simulink model "window_counter_prove"  (R2014b)
settings: Solver=FixedStepDiscrete  StartTime=0.0  StopTime=10.0  FixedStep=0.01  RelTol=1e-3
undefined symbols (not defined in the file): sldvsubsys
libraries: simulink x6, sldvlib x4
settings Model: ModifiedByFormat=Natasha  Creator=Natasha  LastModifiedBy=Natasha
settings DebuggingCC: UnderspecifiedInitializationDetection=Classic  MergeDetectMultiDrivingBlocksExec=none

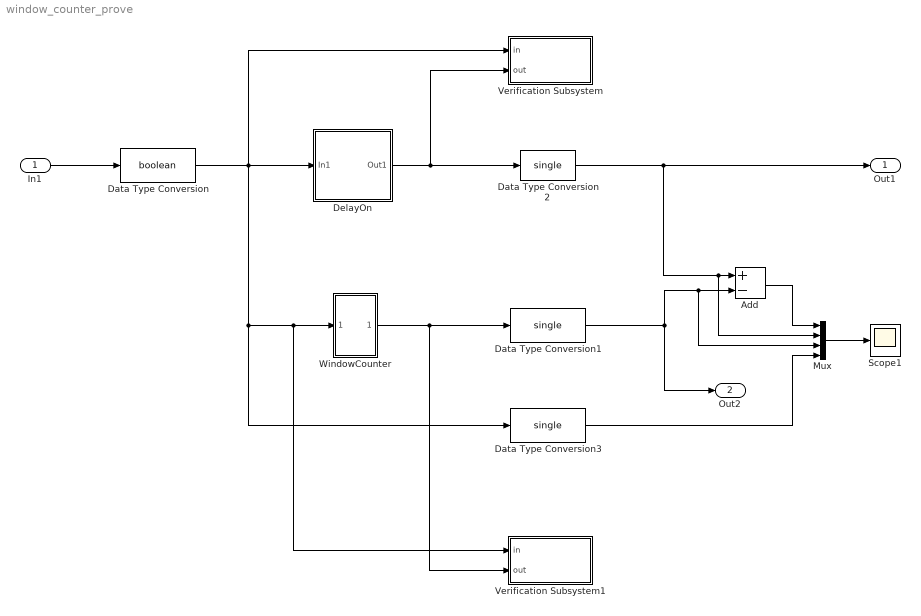
== system window_counter_prove ==
  In1 : Inport
  Add : Sum  Inputs=+-
  Data Type Conversion : DataTypeConversion  OutDataTypeStr=boolean
  Data Type Conversion1 : DataTypeConversion  OutDataTypeStr=single
  Data Type Conversion2 : DataTypeConversion  OutDataTypeStr=single
  Data Type Conversion3 : DataTypeConversion  OutDataTypeStr=single
  DelayOn : Subsystem
  Mux : Mux
  Scope1 : Scope
  Verification Subsystem : Subsystem  Tag=VerificationSubsystem  DisableCoverage=on  LoadFcn=sldvsubsys('check')  TreatAsAtomicUnit=on  SimViewingDevice=on  mask(VerificationSubsystem){}
      mask init:
      | sldvsubsys('maskInit');
      settings: CopyFcn=sldvsubsys('copy');  OpenFcn=open_system(gcb,'force');
      settings: PreSaveFcn=|
      | set_param(gcb,'SimViewingDevice','on');
      | sldvsubsys('check');
      mask Help: helpview(fullfile(docroot,'toolbox','sldv','sldv.map'),'verificationsubsystem')
      mask Display: image(imread('sldvicon_versubsys.png','BackGroundColor',[1 1 1]),'center');
  Verification Subsystem1 : Subsystem  Tag=VerificationSubsystem  DisableCoverage=on  LoadFcn=sldvsubsys('check')  TreatAsAtomicUnit=on  SimViewingDevice=on  mask(VerificationSubsystem){}
      mask init:
      | sldvsubsys('maskInit');
      settings: CopyFcn=sldvsubsys('copy');  OpenFcn=open_system(gcb,'force');
      settings: PreSaveFcn=|
      | set_param(gcb,'SimViewingDevice','on');
      | sldvsubsys('check');
      mask Help: helpview(fullfile(docroot,'toolbox','sldv','sldv.map'),'verificationsubsystem')
      mask Display: image(imread('sldvicon_versubsys.png','BackGroundColor',[1 1 1]),'center');
  WindowCounter : Subsystem
  Out1 : Outport
  Out2 : Outport  Port=2
  wires:
  DelayOn/1(Out1) -> Data Type Conversion2/1, Verification Subsystem/2(out)
  Add/1 -> Mux/1
  Data Type Conversion1/1 -> Out2/1, Mux/3, Add/2
  Data Type Conversion2/1 -> Mux/2, Add/1, Out1/1
  Mux/1 -> Scope1/1
  In1/1 -> Data Type Conversion/1
  WindowCounter/1(Out1) -> Verification Subsystem1/2(out), Data Type Conversion1/1
  Data Type Conversion3/1 -> Mux/4
  Data Type Conversion/1 -> Data Type Conversion3/1, Verification Subsystem1/1(in), WindowCounter/1(In1), DelayOn/1(In1), Verification Subsystem/1(in)

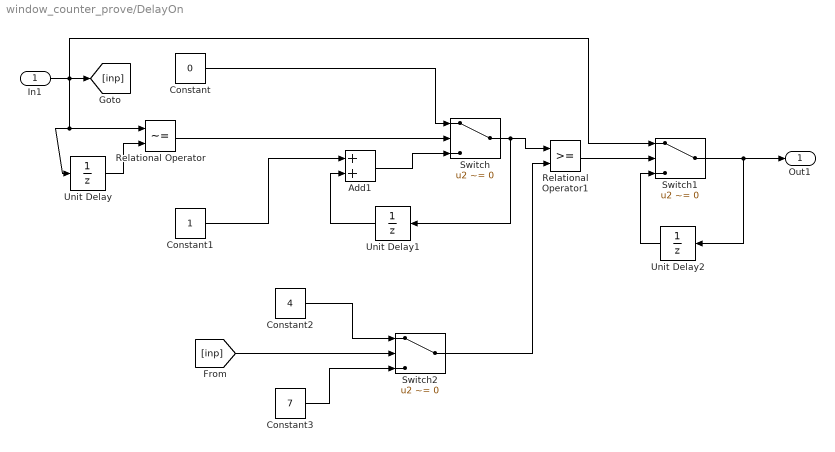
== system window_counter_prove/DelayOn ==
  In1 : Inport
  Add1 : Sum
  Constant : Constant  Value=0
  Constant1 : Constant
  Constant2 : Constant  Value=4
  Constant3 : Constant  Value=7
  Relational Operator : RelationalOperator  Operator=~=  OutDataTypeStr=boolean
  Relational Operator1 : RelationalOperator  OutDataTypeStr=boolean
  Switch : Switch  Criteria=u2 ~= 0
  Switch1 : Switch  Criteria=u2 ~= 0
  Switch2 : Switch  Criteria=u2 ~= 0
  Unit Delay : UnitDelay  InitialCondition=1  SampleTime=-1
  Unit Delay1 : UnitDelay  SampleTime=-1
  Unit Delay2 : UnitDelay  SampleTime=-1
  Out1 : Outport
  wires:
  Unit Delay1/1 -> Add1/2
  Constant2/1 -> Switch2/1
  Constant1/1 -> Add1/1
  Relational Operator/1 -> Switch/2
  Constant/1 -> Switch/1
  Unit Delay/1 -> Relational Operator/2
  Switch1/1 -> Out1/1, Unit Delay2/1
  Unit Delay2/1 -> Switch1/3
  Relational Operator1/1 -> Switch1/2
  Switch/1 -> Unit Delay1/1, Relational Operator1/1
  Constant3/1 -> Switch2/3
  Switch2/1 -> Relational Operator1/2
  Add1/1 -> Switch/3
  [inp] -> Switch2/2
  In1/1 -> Switch1/1, Unit Delay/1, Relational Operator/1, [inp]

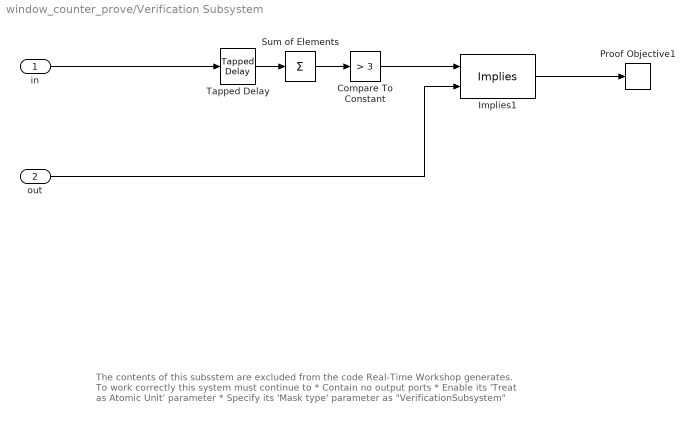
== system window_counter_prove/Verification Subsystem ==
  note: The contents of this subsstem are excluded from the code Real-Time
      | Workshop generates.
      |
      | To work correctly this system must continue to
      | * Contain no output ports
      | * Enable its 'Treat as Atomic Unit' parameter
      | * Specify its 'Mask type' parameter as "VerificationSubsystem"
  in : Inport
  out : Inport  Port=2
  Compare To Constant : simulink/Logic and Bit Operations/Compare To Constant  relop=>  const=3  OutDataTypeStr=boolean
  Implies1 : sldvlib/Verification Utilities/Implies
  Proof Objective1 : sldvlib/Objectives and Constraints/Proof Objective  enabled=on  customAVTBlockType=Proof Objective  intervals=true  dispValues=on  outEnabled=off  enableStopSim=on
      settings: AttributesFormatString=%<intervals>
  Sum of Elements : Sum  Inputs=+
  Tapped Delay : simulink/Discrete/Tapped Delay  vinit=0.0  samptime=-1  NumDelays=10  DelayOrder=Oldest  includeCurrent=off
  wires:
  Compare To Constant/1 -> Implies1/1
  Implies1/1 -> Proof Objective1/1
  Tapped Delay/1 -> Sum of Elements/1
  Sum of Elements/1 -> Compare To Constant/1
  out/1 -> Implies1/2
  in/1 -> Tapped Delay/1

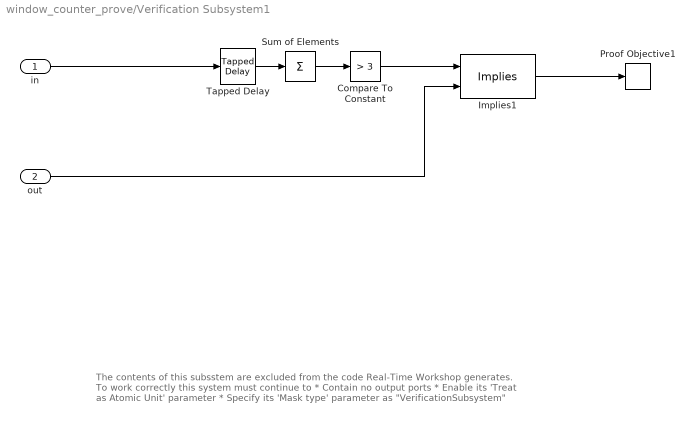
== system window_counter_prove/Verification Subsystem1 ==
  note: The contents of this subsstem are excluded from the code Real-Time
      | Workshop generates.
      |
      | To work correctly this system must continue to
      | * Contain no output ports
      | * Enable its 'Treat as Atomic Unit' parameter
      | * Specify its 'Mask type' parameter as "VerificationSubsystem"
  in : Inport
  out : Inport  Port=2
  Compare To Constant : simulink/Logic and Bit Operations/Compare To Constant  relop=>  const=3  OutDataTypeStr=boolean
  Implies1 : sldvlib/Verification Utilities/Implies
  Proof Objective1 : sldvlib/Objectives and Constraints/Proof Objective  enabled=on  customAVTBlockType=Proof Objective  intervals=true  dispValues=on  outEnabled=off  enableStopSim=on
      settings: AttributesFormatString=%<intervals>
  Sum of Elements : Sum  Inputs=+
  Tapped Delay : simulink/Discrete/Tapped Delay  vinit=0.0  samptime=-1  NumDelays=10  DelayOrder=Oldest  includeCurrent=off
  wires:
  in/1 -> Tapped Delay/1
  out/1 -> Implies1/2
  Sum of Elements/1 -> Compare To Constant/1
  Tapped Delay/1 -> Sum of Elements/1
  Implies1/1 -> Proof Objective1/1
  Compare To Constant/1 -> Implies1/1

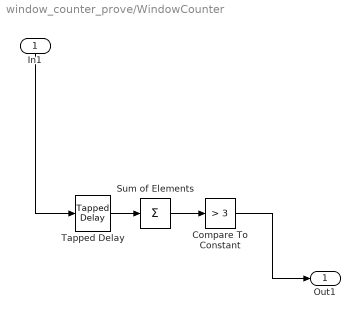
== system window_counter_prove/WindowCounter ==
  In1 : Inport
  Compare To Constant : simulink/Logic and Bit Operations/Compare To Constant  relop=>  const=3  OutDataTypeStr=boolean
  Sum of Elements : Sum  Inputs=+
  Tapped Delay : simulink/Discrete/Tapped Delay  vinit=0.0  samptime=-1  NumDelays=10  DelayOrder=Oldest  includeCurrent=off
  Out1 : Outport
  wires:
  Compare To Constant/1 -> Out1/1
  Tapped Delay/1 -> Sum of Elements/1
  Sum of Elements/1 -> Compare To Constant/1
  In1/1 -> Tapped Delay/1
